simulink model "sampleModel7126_pp_1_1"  (R2018a)
settings: Solver=VariableStepAuto  StartTime=0.0  StopTime=10.0  RelTol=1e-3
undefined symbols (not defined in the file): DiscIntNeverNeededParam
libraries: simulink x367
(part 10 of 12)

== system sampleModel7126_pp_1_1/cfblk287/cfblk4 ==
  emi_718 : Inport
  Action Port : ActionPort  ActionType=then
  cfblk4 : simulink/Discrete/Transfer Fcn Lead or Lag  PoleZ=0.95  ZeroZ=0.75  ICPrevOutput=0.0  ICPrevInput=0.0  DoSatur=off
      settings: SourceProductName=Simulink  SourceProductBaseCode=SL
  emi_719 : Outport
  wires:
  emi_718/1 -> cfblk4/1
  cfblk4/1 -> emi_719/1

== system sampleModel7126_pp_1_1/cfblk287/cfblk6 ==
  emi_753 : Inport
  Action Port : ActionPort  ActionType=then
  cfblk6 : simulink/Discrete/Difference  ICPrevInput=0.0  OutMin=[]  OutMax=[]  OutDataTypeStr=double  OutputDataTypeScalingMode=double  OutDataType=fixdt(1, 16)  OutScaling=2^-10  DoSatur=off
  emi_754 : Outport
  wires:
  emi_753/1 -> cfblk6/1
  cfblk6/1 -> emi_754/1

== system sampleModel7126_pp_1_1/cfblk287/cfblk7 ==
  emi_1674 : Inport
  emi_1675 : Inport  Port=2
  Action Port : ActionPort  ActionType=then
  cfblk7 : Delay  DelayLengthSource=Input port
      settings: InputPortMap=u0,p1
  emi_1676 : Outport
  wires:
  emi_1674/1 -> cfblk7/1
  emi_1675/1 -> cfblk7/2
  cfblk7/1 -> emi_1676/1

== system sampleModel7126_pp_1_1/cfblk287/emi_1677 ==
  Action Port : ActionPort  ActionType=else
  emi_1678 : Assertion

== system sampleModel7126_pp_1_1/cfblk287/emi_720 ==
  Action Port : ActionPort  ActionType=else
  emi_721 : Assertion

== system sampleModel7126_pp_1_1/cfblk287/emi_755 ==
  Action Port : ActionPort  ActionType=else
  emi_756 : Assertion

== system sampleModel7126_pp_1_1/cfblk288/cfblk11 ==
  emi_344 : Inport
  Action Port : ActionPort  ActionType=then
  cfblk11 : simulink/Discrete/Transfer Fcn First Order  PoleZ=0.95  ICPrevOutput=0.0  DoSatur=off
      settings: SourceProductName=Simulink
  emi_345 : Outport
  wires:
  emi_344/1 -> cfblk11/1
  cfblk11/1 -> emi_345/1

== system sampleModel7126_pp_1_1/cfblk288/cfblk3 ==
  emi_1348 : Inport
  Action Port : ActionPort  ActionType=then
  cfblk3 : simulink/Continuous/PID Controller  Controller=PID  TimeDomain=Discrete-time  SampleTime=-1  IntegratorMethod=Forward Euler  FilterMethod=Forward Euler  Form=Parallel  UseFilter=on  ControllerParametersSource=internal  P=1  I=1  D=0  N=100  InitialConditionSource=internal  InitialConditionForIntegrator=0  InitialConditionForFilter=0  ExternalReset=none  LimitOutput=off  UpperSaturationLimit=inf  LowerSaturationLimit=-inf  LinearizeAsGain=off  AntiWindupMode=none  Kb=1  TrackingMode=off  Kt=1  PParamMin=[]  PParamMax=[]  IParamMin=[]  IParamMax=[]  DParamMin=[]  DParamMax=[]  NParamMin=[]  NParamMax=[]  KbParamMin=[]  KbParamMax=[]  KtParamMin=[]  KtParamMax=[]  POutMin=[]  POutMax=[]  IOutMin=[]  IOutMax=[]  DOutMin=[]  DOutMax=[]  NOutMin=[]  NOutMax=[]  KbOutMin=[]  KbOutMax=[]  KtOutMin=[]  KtOutMax=[]  IntegratorOutMin=[]  IntegratorOutMax=[]  FilterOutMin=[]  FilterOutMax=[]  SumOutMin=[]  SumOutMax=[]  SumI1OutMin=[]  SumI1OutMax=[]  SumI2OutMin=[]  SumI2OutMax=[]  SumI3OutMin=[]  SumI3OutMax=[]  SumDOutMin=[]  SumDOutMax=[]  SaturationOutMin=[]  SaturationOutMax=[]  IntegratorContinuousStateAttributes=''  IntegratorStateMustResolveToSignalObject=off  IntegratorRTWStateStorageClass=Auto  FilterContinuousStateAttributes=''  FilterStateMustResolveToSignalObject=off  FilterRTWStateStorageClass=Auto  DifferentiatorICPrevScaledInput=0  DifferentiatorOutMin=[]  DifferentiatorOutMax=[]  FilterDiffOutCoefMin=[]  FilterDiffOutCoefMax=[]  SumDenOutMin=[]  SumDenOutMax=[]  SumNumOutMin=[]  SumNumOutMax=[]  ReciprocalOutMin=[]  ReciprocalOutMax=[]  DivideOutMin=[]  DivideOutMax=[]  TunerSelectOption=Transfer Function Based (PID Tuner App)
  emi_1349 : Outport
  wires:
  emi_1348/1 -> cfblk3/1
  cfblk3/1 -> emi_1349/1

== system sampleModel7126_pp_1_1/cfblk288/emi_1350 ==
  Action Port : ActionPort  ActionType=else
  emi_1351 : Assertion

== system sampleModel7126_pp_1_1/cfblk288/emi_346 ==
  Action Port : ActionPort  ActionType=else
  emi_347 : Assertion

== system sampleModel7126_pp_1_1/cfblk289/cfblk10 ==
  cfblk1 : Inport
  cfblk12 : Inport  Port=2
  Action Port : ActionPort  ActionType=else
  cfblk10 : simulink/Discrete/Transfer Fcn Lead or Lag  PoleZ=0.95  ZeroZ=0.75  ICPrevOutput=0.0  ICPrevInput=0.0  DoSatur=off
      settings: SourceProductName=Simulink  SourceProductBaseCode=SL
  cfblk11 : Delay  DelayLengthSource=Input port
      settings: InputPortMap=u0,p1
  cfblk3 : simulink/Discrete/Transfer Fcn Lead or Lag  PoleZ=0.95  ZeroZ=0.75  ICPrevOutput=0.0  ICPrevInput=0.0  DoSatur=off
      settings: SourceProductName=Simulink  SourceProductBaseCode=SL
  cfblk4 : Subsystem  TreatAsAtomicUnit=on
  cfblk5 : Subsystem  TreatAsAtomicUnit=on
  cfblk6 : Delay  DelayLengthSource=Input port
      settings: InputPortMap=u0,p1
  cfblk7 : Subsystem  TreatAsAtomicUnit=on
  cfblk8 : simulink/Discrete/Difference  ICPrevInput=0.0  OutMin=[]  OutMax=[]  OutDataTypeStr=double  OutputDataTypeScalingMode=double  OutDataType=fixdt(1, 16)  OutScaling=2^-10  DoSatur=off
  cfblk9 : Subsystem  TreatAsAtomicUnit=on
  cyemi_{1097..1107} (11 alike) : DataTypeConversion  OutDataTypeStr=double
  emi_1407 : Subsystem  TreatAsAtomicUnit=on
  emi_{588,978,985,1409} (4 alike) : If  IfExpression=Inf <= u1  SampleTime=[1 0]
  emi_{589,979,986,1410} (4 alike) : DataTypeConversion  OutDataTypeStr=double
  emi_586 : Subsystem  TreatAsAtomicUnit=on
  emi_976 : Subsystem  TreatAsAtomicUnit=on
  emi_983 : Subsystem  TreatAsAtomicUnit=on
  cfblk2 : Outport
  wires:
  cfblk12/1 -> cyemi_1097/1, cyemi_1098/1
  cyemi_1097/1 -> cfblk10/1
  cyemi_1098/1 -> cfblk11/1
  cyemi_1099/1 -> cfblk11/2
  cfblk8/1 -> cyemi_1099/1
  cyemi_1100/1 -> cfblk3/1
  cfblk3/1 -> cyemi_1101/1
  cyemi_1103/1 -> cfblk6/1
  cfblk1/1 -> cyemi_1103/1
  cyemi_1104/1 -> cfblk6/2
  cfblk11/1 -> cyemi_1105/1, emi_979/1, emi_986/1, emi_1410/1
  cyemi_1106/1 -> cfblk8/1
  cfblk10/1 -> cyemi_1106/1
  cfblk6/1 -> cyemi_1107/1, emi_589/1
  cyemi_1107/1 -> cfblk9/1(emi_584)
  cfblk9/1(emi_585) -> cyemi_1102/1
  emi_588/1 -> cfblk9/Action
  emi_588/2 -> emi_586/Action
  emi_589/1 -> emi_588/1
  cyemi_1102/1 -> cfblk5/1(emi_974)
  cfblk5/1(emi_975) -> cyemi_1100/1
  emi_978/1 -> cfblk5/Action
  emi_978/2 -> emi_976/Action
  emi_979/1 -> emi_978/1
  cyemi_1101/1 -> cfblk4/1(emi_981)
  cfblk4/1(emi_982) -> cfblk2/1
  emi_985/1 -> cfblk4/Action
  emi_985/2 -> emi_983/Action
  emi_986/1 -> emi_985/1
  cyemi_1105/1 -> cfblk7/1(emi_1405)
  cfblk7/1(emi_1406) -> cyemi_1104/1
  emi_1409/1 -> cfblk7/Action
  emi_1409/2 -> emi_1407/Action
  emi_1410/1 -> emi_1409/1

== system sampleModel7126_pp_1_1/cfblk289/cfblk11 ==
  emi_1124 : Inport
  Action Port : ActionPort  ActionType=then
  cfblk11 : Delay
  emi_1125 : Outport
  wires:
  emi_1124/1 -> cfblk11/1
  cfblk11/1 -> emi_1125/1

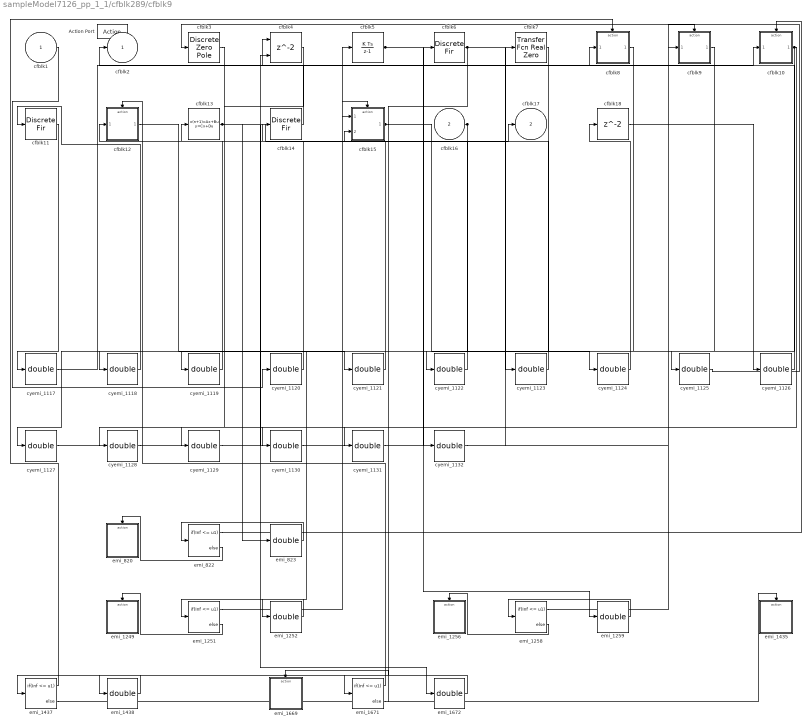
== system sampleModel7126_pp_1_1/cfblk289/cfblk9 ==
  cfblk1 : Inport
  cfblk16 : Inport  Port=2
  Action Port : ActionPort  ActionType=then
  cfblk10 : Subsystem  TreatAsAtomicUnit=on
  cfblk11 : DiscreteFir
  cfblk12 : Subsystem  TreatAsAtomicUnit=on
  cfblk13 : DiscreteStateSpace  SampleTime=-1
  cfblk14 : DiscreteFir
  cfblk15 : Subsystem  TreatAsAtomicUnit=on
  cfblk18 : Delay
  cfblk3 : DiscreteZeroPole  Poles=[0 0.5]  Gain=1  SampleTime=-1
  cfblk4 : Delay  ShowEnablePort=on
      settings: InputPortMap=u0,e6
  cfblk5 : DiscreteIntegrator  SampleTime=-1  OutDataTypeStr=double  ICPrevOutput=DiscIntNeverNeededParam  ICPrevScaledInput=DiscIntNeverNeededParam
  cfblk6 : DiscreteFir
  cfblk7 : simulink/Discrete/Transfer Fcn Real Zero  ZeroZ=0.75  ICPrevInput=0.0  DoSatur=off
      settings: SourceProductName=Simulink  SourceProductBaseCode=SL
  cfblk8 : Subsystem  TreatAsAtomicUnit=on
  cfblk9 : Subsystem  TreatAsAtomicUnit=on
  cyemi_{1117..1132} (16 alike) : DataTypeConversion  OutDataTypeStr=double
  emi_1249 : Subsystem  TreatAsAtomicUnit=on
  emi_1251 : If  IfExpression=Inf <= u1  SampleTime=[1 0]
  emi_{823,1252,1259,1438,1672} (5 alike) : DataTypeConversion  OutDataTypeStr=double
  emi_1256 : Subsystem  TreatAsAtomicUnit=on
  emi_1258 : If  IfExpression=Inf <= u1  SampleTime=[0 1]
  emi_1435 : Subsystem  TreatAsAtomicUnit=on
  emi_1437 : If  IfExpression=Inf <= u1  SampleTime=[1 0]
  emi_1669 : Subsystem  TreatAsAtomicUnit=on
  emi_1671 : If  IfExpression=Inf <= u1  SampleTime=[1 0]
  emi_820 : Subsystem  TreatAsAtomicUnit=on
  emi_822 : If  IfExpression=Inf <= u1
  cfblk2 : Outport
  cfblk17 : Outport  Port=2
  wires:
  cfblk16/1 -> cyemi_1127/1, cyemi_1130/1
  cfblk14/1 -> cfblk2/1
  cfblk13/1 -> cfblk17/1, emi_823/1, emi_1672/1
  cfblk11/1 -> cyemi_1117/1
  cyemi_1118/1 -> cfblk11/1
  cfblk7/1 -> cyemi_1118/1
  cfblk3/1 -> cyemi_1119/1
  cyemi_1120/1 -> cfblk13/1
  cfblk1/1 -> cyemi_1120/1
  cyemi_1121/1 -> cfblk14/1
  cfblk6/1 -> cyemi_1123/1, emi_1438/1
  cyemi_1124/1 -> cfblk18/1
  cyemi_1125/1 -> cfblk3/1
  cyemi_1126/1 -> cfblk4/1
  cfblk18/1 -> cyemi_1126/1
  cyemi_1127/1 -> cfblk4/2
  cyemi_1128/1 -> cfblk5/1
  cyemi_1129/1 -> cfblk6/1
  cfblk4/1 -> cyemi_1129/1
  cyemi_1130/1 -> cfblk7/1
  cfblk5/1 -> cyemi_1132/1, emi_1259/1
  cyemi_1117/1 -> cfblk10/1(emi_818)
  cfblk10/1(emi_819) -> cyemi_1131/1, emi_1252/1
  emi_822/1 -> cfblk10/Action
  emi_822/2 -> emi_820/Action
  emi_823/1 -> emi_822/1
  cyemi_1122/1 -> cfblk15/1(emi_1246)
  cyemi_1123/1 -> cfblk15/2(emi_1247)
  cfblk15/1(emi_1248) -> cyemi_1128/1, cyemi_1124/1
  emi_1251/1 -> cfblk15/Action
  emi_1251/2 -> emi_1249/Action
  emi_1252/1 -> emi_1251/1
  cyemi_1132/1 -> cfblk9/1(emi_1254)
  cfblk9/1(emi_1255) -> cyemi_1125/1
  emi_1258/1 -> cfblk9/Action
  emi_1258/2 -> emi_1256/Action
  emi_1259/1 -> emi_1258/1
  cyemi_1131/1 -> cfblk8/1(emi_1433)
  cfblk8/1(emi_1434) -> cyemi_1122/1
  emi_1437/1 -> cfblk8/Action
  emi_1437/2 -> emi_1435/Action
  emi_1438/1 -> emi_1437/1
  cyemi_1119/1 -> cfblk12/1(emi_1667)
  cfblk12/1(emi_1668) -> cyemi_1121/1
  emi_1671/1 -> cfblk12/Action
  emi_1671/2 -> emi_1669/Action
  emi_1672/1 -> emi_1671/1

== system sampleModel7126_pp_1_1/cfblk289/emi_1126 ==
  Action Port : ActionPort  ActionType=else
  emi_1127 : Assertion

== system sampleModel7126_pp_1_1/cfblk290/cfblk3 ==
  emi_1725 : Inport
  Action Port : ActionPort  ActionType=then
  cfblk3 : DiscreteTransferFcn
  emi_1726 : Outport
  wires:
  emi_1725/1 -> cfblk3/1
  cfblk3/1 -> emi_1726/1

== system sampleModel7126_pp_1_1/cfblk290/cfblk5 ==
  emi_1239 : Inport
  Action Port : ActionPort  ActionType=then
  cfblk5 : DiscreteFilter
  emi_1240 : Outport
  wires:
  emi_1239/1 -> cfblk5/1
  cfblk5/1 -> emi_1240/1

== system sampleModel7126_pp_1_1/cfblk290/cfblk6 ==
  emi_1869 : Inport
  emi_1870 : Inport  Port=2
  Action Port : ActionPort  ActionType=then
  cfblk6 : simulink/Continuous/PID Controller (2DOF)  Controller=PID  TimeDomain=Discrete-time  SampleTime=-1  IntegratorMethod=Forward Euler  FilterMethod=Forward Euler  Form=Parallel  UseFilter=on  ControllerParametersSource=internal  P=1  I=1  D=0  N=100  b=1  c=1  InitialConditionSource=internal  InitialConditionForIntegrator=0  InitialConditionForFilter=0  ExternalReset=none  LimitOutput=off  UpperSaturationLimit=inf  LowerSaturationLimit=-inf  LinearizeAsGain=off  AntiWindupMode=none  Kb=1  TrackingMode=off  Kt=1  PParamMin=[]  PParamMax=[]  IParamMin=[]  IParamMax=[]  DParamMin=[]  DParamMax=[]  NParamMin=[]  NParamMax=[]  bParamMin=[]  bParamMax=[]  cParamMin=[]  cParamMax=[]  KbParamMin=[]  KbParamMax=[]  KtParamMin=[]  KtParamMax=[]  POutMin=[]  POutMax=[]  IOutMin=[]  IOutMax=[]  DOutMin=[]  DOutMax=[]  NOutMin=[]  NOutMax=[]  bOutMin=[]  bOutMax=[]  cOutMin=[]  cOutMax=[]  KbOutMin=[]  KbOutMax=[]  KtOutMin=[]  KtOutMax=[]  IntegratorOutMin=[]  IntegratorOutMax=[]  FilterOutMin=[]  FilterOutMax=[]  SumOutMin=[]  SumOutMax=[]  Sum1OutMin=[]  Sum1OutMax=[]  Sum2OutMin=[]  Sum2OutMax=[]  Sum3OutMin=[]  Sum3OutMax=[]  SumI1OutMin=[]  SumI1OutMax=[]  SumI2OutMin=[]  SumI2OutMax=[]  SumI3OutMin=[]  SumI3OutMax=[]  SumDOutMin=[]  SumDOutMax=[]  SaturationOutMin=[]  SaturationOutMax=[]  IntegratorContinuousStateAttributes=''  IntegratorStateMustResolveToSignalObject=off  IntegratorRTWStateStorageClass=Auto  FilterContinuousStateAttributes=''  FilterStateMustResolveToSignalObject=off  FilterRTWStateStorageClass=Auto  DifferentiatorICPrevScaledInput=0  DifferentiatorOutMin=[]  DifferentiatorOutMax=[]  FilterDiffOutCoefMin=[]  FilterDiffOutCoefMax=[]  SumDenOutMin=[]  SumDenOutMax=[]  SumNumOutMin=[]  SumNumOutMax=[]  ReciprocalOutMin=[]  ReciprocalOutMax=[]  DivideOutMin=[]  DivideOutMax=[]  TunerSelectOption=Transfer Function Based (PID Tuner App)
  emi_1871 : Outport
  wires:
  emi_1869/1 -> cfblk6/1
  emi_1870/1 -> cfblk6/2
  cfblk6/1 -> emi_1871/1

== system sampleModel7126_pp_1_1/cfblk290/cfblk7 ==
  emi_1383 : Inport
  Action Port : ActionPort  ActionType=then
  cfblk7 : DiscreteFilter
  emi_1384 : Outport
  wires:
  emi_1383/1 -> cfblk7/1
  cfblk7/1 -> emi_1384/1

== system sampleModel7126_pp_1_1/cfblk290/cfblk8 ==
  emi_1152 : Inport
  Action Port : ActionPort  ActionType=then
  cfblk8 : Delay
  emi_1153 : Outport
  wires:
  emi_1152/1 -> cfblk8/1
  cfblk8/1 -> emi_1153/1

== system sampleModel7126_pp_1_1/cfblk290/emi_1154 ==
  Action Port : ActionPort  ActionType=else
  emi_1155 : Assertion

== system sampleModel7126_pp_1_1/cfblk290/emi_1241 ==
  Action Port : ActionPort  ActionType=else
  emi_1242 : Assertion

== system sampleModel7126_pp_1_1/cfblk290/emi_1385 ==
  Action Port : ActionPort  ActionType=else
  emi_1386 : Assertion

== system sampleModel7126_pp_1_1/cfblk290/emi_1727 ==
  Action Port : ActionPort  ActionType=else
  emi_1728 : Assertion

== system sampleModel7126_pp_1_1/cfblk290/emi_1872 ==
  Action Port : ActionPort  ActionType=else
  emi_1873 : Assertion

== system sampleModel7126_pp_1_1/cfblk291/cfblk6 ==
  emi_429 : Inport
  emi_430 : Inport  Port=2
  Action Port : ActionPort  ActionType=then
  cfblk6 : Delay  ShowEnablePort=on
      settings: InputPortMap=u0,e6
  emi_431 : Outport
  wires:
  emi_429/1 -> cfblk6/1
  emi_430/1 -> cfblk6/2
  cfblk6/1 -> emi_431/1

== system sampleModel7126_pp_1_1/cfblk291/emi_432 ==
  Action Port : ActionPort  ActionType=else
  emi_433 : Assertion

== system sampleModel7126_pp_1_1/cfblk292/cfblk14 ==
  cfblk1 : Inport
  Action Port : ActionPort  ActionType=then
  cfblk3 : Subsystem  TreatAsAtomicUnit=on
  cfblk4 : Subsystem  TreatAsAtomicUnit=on
  cfblk5 : simulink/Discrete/Tapped Delay  vinit=0.0  samptime=-1  NumDelays=1  DelayOrder=Oldest  includeCurrent=off
  cfblk6 : simulink/Continuous/PID Controller (2DOF)  Controller=PID  TimeDomain=Discrete-time  SampleTime=-1  IntegratorMethod=Forward Euler  FilterMethod=Forward Euler  Form=Parallel  UseFilter=on  ControllerParametersSource=internal  P=1  I=1  D=0  N=100  b=1  c=1  InitialConditionSource=internal  InitialConditionForIntegrator=0  InitialConditionForFilter=0  ExternalReset=none  LimitOutput=off  UpperSaturationLimit=inf  LowerSaturationLimit=-inf  LinearizeAsGain=off  AntiWindupMode=none  Kb=1  TrackingMode=off  Kt=1  PParamMin=[]  PParamMax=[]  IParamMin=[]  IParamMax=[]  DParamMin=[]  DParamMax=[]  NParamMin=[]  NParamMax=[]  bParamMin=[]  bParamMax=[]  cParamMin=[]  cParamMax=[]  KbParamMin=[]  KbParamMax=[]  KtParamMin=[]  KtParamMax=[]  POutMin=[]  POutMax=[]  IOutMin=[]  IOutMax=[]  DOutMin=[]  DOutMax=[]  NOutMin=[]  NOutMax=[]  bOutMin=[]  bOutMax=[]  cOutMin=[]  cOutMax=[]  KbOutMin=[]  KbOutMax=[]  KtOutMin=[]  KtOutMax=[]  IntegratorOutMin=[]  IntegratorOutMax=[]  FilterOutMin=[]  FilterOutMax=[]  SumOutMin=[]  SumOutMax=[]  Sum1OutMin=[]  Sum1OutMax=[]  Sum2OutMin=[]  Sum2OutMax=[]  Sum3OutMin=[]  Sum3OutMax=[]  SumI1OutMin=[]  SumI1OutMax=[]  SumI2OutMin=[]  SumI2OutMax=[]  SumI3OutMin=[]  SumI3OutMax=[]  SumDOutMin=[]  SumDOutMax=[]  SaturationOutMin=[]  SaturationOutMax=[]  IntegratorContinuousStateAttributes=''  IntegratorStateMustResolveToSignalObject=off  IntegratorRTWStateStorageClass=Auto  FilterContinuousStateAttributes=''  FilterStateMustResolveToSignalObject=off  FilterRTWStateStorageClass=Auto  DifferentiatorICPrevScaledInput=0  DifferentiatorOutMin=[]  DifferentiatorOutMax=[]  FilterDiffOutCoefMin=[]  FilterDiffOutCoefMax=[]  SumDenOutMin=[]  SumDenOutMax=[]  SumNumOutMin=[]  SumNumOutMax=[]  ReciprocalOutMin=[]  ReciprocalOutMax=[]  DivideOutMin=[]  DivideOutMax=[]  TunerSelectOption=Transfer Function Based (PID Tuner App)
  cfblk8 : Delay
  cfblk9 : Delay
  cyemi_{1158..1164} (7 alike) : DataTypeConversion  OutDataTypeStr=double
  emi_1428 : Subsystem  TreatAsAtomicUnit=on
  emi_1430 : If  IfExpression=Inf <= u1
  emi_1431 : DataTypeConversion  OutDataTypeStr=double
  emi_353 : Subsystem  TreatAsAtomicUnit=on
  emi_355 : If  IfExpression=Inf <= u1  SampleTime=[1 0]
  emi_356 : DataTypeConversion  OutDataTypeStr=double
  cfblk2 : Outport
  cfblk7 : Outport  Port=2
  wires:
  cfblk5/1 -> cyemi_1163/1, cyemi_1164/1
  cfblk8/1 -> cyemi_1158/1, emi_356/1, emi_1431/1
  cfblk1/1 -> cyemi_1159/1
  cyemi_1160/1 -> cfblk5/1
  cfblk6/1 -> cyemi_1160/1
  cyemi_1161/1 -> cfblk6/1
  cfblk9/1 -> cyemi_1161/1
  cyemi_1162/1 -> cfblk6/2
  cyemi_1163/1 -> cfblk8/1
  cyemi_1164/1 -> cfblk9/1
  cyemi_1159/1 -> cfblk4/1(emi_351)
  cfblk4/1(emi_352) -> cfblk7/1
  emi_355/1 -> cfblk4/Action
  emi_355/2 -> emi_353/Action
  emi_356/1 -> emi_355/1
  cyemi_1158/1 -> cfblk3/1(emi_1426)
  cfblk3/1(emi_1427) -> cyemi_1162/1, cfblk2/1
  emi_1430/1 -> cfblk3/Action
  emi_1430/2 -> emi_1428/Action
  emi_1431/1 -> emi_1430/1

== system sampleModel7126_pp_1_1/cfblk292/cfblk15 ==
  cfblk1 : Inport
  cfblk8 : Inport  Port=2
  cfblk9 : Inport  Port=3
  cfblk10 : Inport  Port=4
  Action Port : ActionPort  ActionType=else
  cfblk13 : Subsystem  TreatAsAtomicUnit=on
  cfblk3 : Subsystem  TreatAsAtomicUnit=on
  cfblk4 : UnitDelay  SampleTime=-1
  cfblk5 : Subsystem  TreatAsAtomicUnit=on
  cfblk6 : Subsystem  TreatAsAtomicUnit=on
  cfblk7 : DiscreteTransferFcn
  cyemi_{1169..1175} (7 alike) : DataTypeConversion  OutDataTypeStr=double
  emi_1414 : Subsystem  TreatAsAtomicUnit=on
  emi_1416 : If  IfExpression=0 <= u1
  emi_{458,1417,1738,1767} (4 alike) : DataTypeConversion  OutDataTypeStr=double
  emi_1735 : Subsystem  TreatAsAtomicUnit=on
  emi_1737 : If  IfExpression=0 <= u1  SampleTime=[1 0]
  emi_1764 : Subsystem  TreatAsAtomicUnit=on
  emi_1766 : If  IfExpression=0 <= u1  SampleTime=[1 0]
  emi_455 : Subsystem  TreatAsAtomicUnit=on
  emi_457 : If  IfExpression=0 <= u1
  cfblk2 : Outport
  cfblk11 : Outport  Port=2
  cfblk12 : Outport  Port=3
  wires:
  cfblk9/1 -> cfblk12/1
  cfblk8/1 -> cfblk2/1
  cfblk4/1 -> cfblk11/1
  cfblk1/1 -> cyemi_1170/1
  cyemi_1171/1 -> cfblk4/1
  cfblk7/1 -> cyemi_1171/1, emi_1738/1
  cyemi_1175/1 -> cfblk7/1
  cfblk10/1 -> cyemi_1175/1
  cyemi_1170/1 -> cfblk3/1(emi_453)
  cfblk3/1(emi_454) -> cyemi_1174/1
  emi_457/1 -> cfblk3/Action
  emi_457/2 -> emi_455/Action
  emi_458/1 -> emi_457/1
  cyemi_1169/1 -> cfblk13/1(emi_1412)
  cfblk13/1(emi_1413) -> emi_458/1, cyemi_1173/1, emi_1767/1
  emi_1416/1 -> cfblk13/Action
  emi_1416/2 -> emi_1414/Action
  emi_1417/1 -> emi_1416/1
  cyemi_1173/1 -> cfblk6/1(emi_1732)
  cyemi_1174/1 -> cfblk6/2(emi_1733)
  cfblk6/1(emi_1734) -> cyemi_1172/1
  emi_1737/1 -> cfblk6/Action
  emi_1737/2 -> emi_1735/Action
  emi_1738/1 -> emi_1737/1
  cyemi_1172/1 -> cfblk5/1(emi_1762)
  cfblk5/1(emi_1763) -> emi_1417/1, cyemi_1169/1
  emi_1766/1 -> cfblk5/Action
  emi_1766/2 -> emi_1764/Action
  emi_1767/1 -> emi_1766/1

== system sampleModel7126_pp_1_1/cfblk292/cfblk16 ==
  emi_301 : Inport
  Action Port : ActionPort  ActionType=then
  cfblk16 : Delay
  emi_302 : Outport
  wires:
  emi_301/1 -> cfblk16/1
  cfblk16/1 -> emi_302/1

== system sampleModel7126_pp_1_1/cfblk292/cfblk6 ==
  emi_1110 : Inport
  Action Port : ActionPort  ActionType=then
  cfblk6 : simulink/Discrete/Tapped Delay  vinit=0.0  samptime=-1  NumDelays=1  DelayOrder=Oldest  includeCurrent=off
  emi_1111 : Outport
  wires:
  emi_1110/1 -> cfblk6/1
  cfblk6/1 -> emi_1111/1

== system sampleModel7126_pp_1_1/cfblk292/emi_1112 ==
  Action Port : ActionPort  ActionType=else
  emi_1113 : Assertion

== system sampleModel7126_pp_1_1/cfblk292/emi_303 ==
  Action Port : ActionPort  ActionType=else
  emi_304 : Assertion

== system sampleModel7126_pp_1_1/cfblk293/cfblk10 ==
  emi_2173 : Inport
  Action Port : ActionPort  ActionType=then
  cfblk10 : Delay
  emi_2174 : Outport
  wires:
  emi_2173/1 -> cfblk10/1
  cfblk10/1 -> emi_2174/1

== system sampleModel7126_pp_1_1/cfblk293/cfblk12 ==
  emi_117 : Inport
  Action Port : ActionPort  ActionType=then
  cfblk12 : Delay
  emi_118 : Outport
  wires:
  emi_117/1 -> cfblk12/1
  cfblk12/1 -> emi_118/1

== system sampleModel7126_pp_1_1/cfblk293/cfblk4 ==
  emi_322 : Inport
  emi_323 : Inport  Port=2
  Action Port : ActionPort  ActionType=then
  cfblk4 : Delay  ShowEnablePort=on
      settings: InputPortMap=u0,e6
  emi_324 : Outport
  wires:
  emi_322/1 -> cfblk4/1
  emi_323/1 -> cfblk4/2
  cfblk4/1 -> emi_324/1

== system sampleModel7126_pp_1_1/cfblk293/cfblk8 ==
  emi_294 : Inport
  Action Port : ActionPort  ActionType=then
  cfblk8 : simulink/Discrete/Transfer Fcn First Order  PoleZ=0.95  ICPrevOutput=0.0  DoSatur=off
      settings: SourceProductName=Simulink
  emi_295 : Outport
  wires:
  emi_294/1 -> cfblk8/1
  cfblk8/1 -> emi_295/1

== system sampleModel7126_pp_1_1/cfblk293/emi_119 ==
  Action Port : ActionPort  ActionType=else
  emi_120 : Assertion

== system sampleModel7126_pp_1_1/cfblk293/emi_2175 ==
  Action Port : ActionPort  ActionType=else
  emi_2176 : Assertion

== system sampleModel7126_pp_1_1/cfblk293/emi_296 ==
  Action Port : ActionPort  ActionType=else
  emi_297 : Assertion

== system sampleModel7126_pp_1_1/cfblk293/emi_325 ==
  Action Port : ActionPort  ActionType=else
  emi_326 : Assertion

== system sampleModel7126_pp_1_1/cfblk294/cfblk3 ==
  emi_1390 : Inport
  emi_1391 : Inport  Port=2
  Action Port : ActionPort  ActionType=then
  cfblk3 : Delay  DelayLengthSource=Input port
      settings: InputPortMap=u0,p1
  emi_1392 : Outport
  wires:
  emi_1390/1 -> cfblk3/1
  emi_1391/1 -> cfblk3/2
  cfblk3/1 -> emi_1392/1

== system sampleModel7126_pp_1_1/cfblk294/cfblk7 ==
  emi_1188 : Inport
  Action Port : ActionPort  ActionType=then
  cfblk7 : Delay
  emi_1189 : Outport
  wires:
  emi_1188/1 -> cfblk7/1
  cfblk7/1 -> emi_1189/1

== system sampleModel7126_pp_1_1/cfblk294/emi_1190 ==
  Action Port : ActionPort  ActionType=else
  emi_1191 : Assertion

== system sampleModel7126_pp_1_1/cfblk294/emi_1393 ==
  Action Port : ActionPort  ActionType=else
  emi_1394 : Assertion

== system sampleModel7126_pp_1_1/cfblk295/cfblk13 ==
  cfblk1 : Inport
  cfblk15 : Inport  Port=2
  cfblk16 : Inport  Port=3
  cfblk17 : Inport  Port=4
  Action Port : ActionPort  ActionType=then
  cfblk10 : simulink/Discrete/Transfer Fcn Real Zero  ZeroZ=0.75  ICPrevInput=0.0  DoSatur=off
      settings: SourceProductName=Simulink  SourceProductBaseCode=SL
  cfblk11 : DiscreteStateSpace  SampleTime=-1
  cfblk12 : DiscreteFir
  cfblk13 : Delay  DelayLengthSource=Input port
      settings: InputPortMap=u0,p1
  cfblk14 : DiscreteFir
  cfblk3 : simulink/Continuous/PID Controller  Controller=PID  TimeDomain=Discrete-time  SampleTime=-1  IntegratorMethod=Forward Euler  FilterMethod=Forward Euler  Form=Parallel  UseFilter=on  ControllerParametersSource=internal  P=1  I=1  D=0  N=100  InitialConditionSource=internal  InitialConditionForIntegrator=0  InitialConditionForFilter=0  ExternalReset=none  LimitOutput=off  UpperSaturationLimit=inf  LowerSaturationLimit=-inf  LinearizeAsGain=off  AntiWindupMode=none  Kb=1  TrackingMode=off  Kt=1  PParamMin=[]  PParamMax=[]  IParamMin=[]  IParamMax=[]  DParamMin=[]  DParamMax=[]  NParamMin=[]  NParamMax=[]  KbParamMin=[]  KbParamMax=[]  KtParamMin=[]  KtParamMax=[]  POutMin=[]  POutMax=[]  IOutMin=[]  IOutMax=[]  DOutMin=[]  DOutMax=[]  NOutMin=[]  NOutMax=[]  KbOutMin=[]  KbOutMax=[]  KtOutMin=[]  KtOutMax=[]  IntegratorOutMin=[]  IntegratorOutMax=[]  FilterOutMin=[]  FilterOutMax=[]  SumOutMin=[]  SumOutMax=[]  SumI1OutMin=[]  SumI1OutMax=[]  SumI2OutMin=[]  SumI2OutMax=[]  SumI3OutMin=[]  SumI3OutMax=[]  SumDOutMin=[]  SumDOutMax=[]  SaturationOutMin=[]  SaturationOutMax=[]  IntegratorContinuousStateAttributes=''  IntegratorStateMustResolveToSignalObject=off  IntegratorRTWStateStorageClass=Auto  FilterContinuousStateAttributes=''  FilterStateMustResolveToSignalObject=off  FilterRTWStateStorageClass=Auto  DifferentiatorICPrevScaledInput=0  DifferentiatorOutMin=[]  DifferentiatorOutMax=[]  FilterDiffOutCoefMin=[]  FilterDiffOutCoefMax=[]  SumDenOutMin=[]  SumDenOutMax=[]  SumNumOutMin=[]  SumNumOutMax=[]  ReciprocalOutMin=[]  ReciprocalOutMax=[]  DivideOutMin=[]  DivideOutMax=[]  TunerSelectOption=Transfer Function Based (PID Tuner App)
  cfblk4 : simulink/Discrete/Tapped Delay  vinit=0.0  samptime=-1  NumDelays=1  DelayOrder=Oldest  includeCurrent=off
  cfblk5 : Subsystem  TreatAsAtomicUnit=on
  cfblk6 : simulink/Discrete/Difference  ICPrevInput=0.0  OutMin=[]  OutMax=[]  OutDataTypeStr=double  OutputDataTypeScalingMode=double  OutDataType=fixdt(1, 16)  OutScaling=2^-10  DoSatur=off
  cfblk7 : simulink/Continuous/PID Controller (2DOF)  Controller=PID  TimeDomain=Discrete-time  SampleTime=-1  IntegratorMethod=Forward Euler  FilterMethod=Forward Euler  Form=Parallel  UseFilter=on  ControllerParametersSource=internal  P=1  I=1  D=0  N=100  b=1  c=1  InitialConditionSource=internal  InitialConditionForIntegrator=0  InitialConditionForFilter=0  ExternalReset=none  LimitOutput=off  UpperSaturationLimit=inf  LowerSaturationLimit=-inf  LinearizeAsGain=off  AntiWindupMode=none  Kb=1  TrackingMode=off  Kt=1  PParamMin=[]  PParamMax=[]  IParamMin=[]  IParamMax=[]  DParamMin=[]  DParamMax=[]  NParamMin=[]  NParamMax=[]  bParamMin=[]  bParamMax=[]  cParamMin=[]  cParamMax=[]  KbParamMin=[]  KbParamMax=[]  KtParamMin=[]  KtParamMax=[]  POutMin=[]  POutMax=[]  IOutMin=[]  IOutMax=[]  DOutMin=[]  DOutMax=[]  NOutMin=[]  NOutMax=[]  bOutMin=[]  bOutMax=[]  cOutMin=[]  cOutMax=[]  KbOutMin=[]  KbOutMax=[]  KtOutMin=[]  KtOutMax=[]  IntegratorOutMin=[]  IntegratorOutMax=[]  FilterOutMin=[]  FilterOutMax=[]  SumOutMin=[]  SumOutMax=[]  Sum1OutMin=[]  Sum1OutMax=[]  Sum2OutMin=[]  Sum2OutMax=[]  Sum3OutMin=[]  Sum3OutMax=[]  SumI1OutMin=[]  SumI1OutMax=[]  SumI2OutMin=[]  SumI2OutMax=[]  SumI3OutMin=[]  SumI3OutMax=[]  SumDOutMin=[]  SumDOutMax=[]  SaturationOutMin=[]  SaturationOutMax=[]  IntegratorContinuousStateAttributes=''  IntegratorStateMustResolveToSignalObject=off  IntegratorRTWStateStorageClass=Auto  FilterContinuousStateAttributes=''  FilterStateMustResolveToSignalObject=off  FilterRTWStateStorageClass=Auto  DifferentiatorICPrevScaledInput=0  DifferentiatorOutMin=[]  DifferentiatorOutMax=[]  FilterDiffOutCoefMin=[]  FilterDiffOutCoefMax=[]  SumDenOutMin=[]  SumDenOutMax=[]  SumNumOutMin=[]  SumNumOutMax=[]  ReciprocalOutMin=[]  ReciprocalOutMax=[]  DivideOutMin=[]  DivideOutMax=[]  TunerSelectOption=Transfer Function Based (PID Tuner App)
  cfblk8 : simulink/Discrete/Transfer Fcn Real Zero  ZeroZ=0.75  ICPrevInput=0.0  DoSatur=off
      settings: SourceProductName=Simulink  SourceProductBaseCode=SL
  cfblk9 : simulink/Discrete/Tapped Delay  vinit=0.0  samptime=-1  NumDelays=1  DelayOrder=Oldest  includeCurrent=off
  cyemi_{1224..1237} (14 alike) : DataTypeConversion  OutDataTypeStr=double
  emi_990 : Subsystem  TreatAsAtomicUnit=on
  emi_992 : If  IfExpression=Inf <= u1  SampleTime=[1 0]
  emi_993 : DataTypeConversion  OutDataTypeStr=double
  cfblk2 : Outport
  wires:
  cfblk4/1 -> cfblk2/1
  cyemi_1224/1 -> cfblk10/1
  cfblk1/1 -> cyemi_1224/1
  cyemi_1225/1 -> cfblk11/1
  cfblk14/1 -> cyemi_1225/1
  cyemi_1226/1 -> cfblk12/1
  cfblk11/1 -> cyemi_1226/1
  cyemi_1227/1 -> cfblk13/1
  cfblk17/1 -> cyemi_1227/1
  cyemi_1228/1 -> cfblk13/2
  cyemi_1229/1 -> cfblk14/1
  cfblk16/1 -> cyemi_1229/1
  cyemi_1230/1 -> cfblk3/1
  cfblk10/1 -> cyemi_1230/1
  cyemi_1231/1 -> cfblk4/1
  cfblk8/1 -> cyemi_1231/1
  cfblk15/1 -> cyemi_1232/1
  cyemi_1233/1 -> cfblk6/1
  cfblk9/1 -> cyemi_1233/1
  cyemi_1234/1 -> cfblk7/1
  cfblk6/1 -> cyemi_1234/1
  cyemi_1235/1 -> cfblk7/2
  cfblk13/1 -> cyemi_1235/1, emi_993/1
  cyemi_1236/1 -> cfblk8/1
  cfblk7/1 -> cyemi_1236/1
  cyemi_1237/1 -> cfblk9/1
  cfblk12/1 -> cyemi_1237/1
  cyemi_1232/1 -> cfblk5/1(emi_988)
  cfblk5/1(emi_989) -> cyemi_1228/1
  emi_992/1 -> cfblk5/Action
  emi_992/2 -> emi_990/Action
  emi_993/1 -> emi_992/1

== system sampleModel7126_pp_1_1/cfblk295/cfblk14 ==
  cfblk1 : Inport
  cfblk14 : Inport  Port=2
  cfblk15 : Inport  Port=3
  Action Port : ActionPort  ActionType=else
  cfblk10 : UnitDelay  SampleTime=-1
  cfblk11 : Subsystem  TreatAsAtomicUnit=on
  cfblk12 : Subsystem  TreatAsAtomicUnit=on
  cfblk13 : DiscreteZeroPole  Poles=[0 0.5]  Gain=1  SampleTime=-1
  cfblk16 : Delay
  cfblk3 : DiscreteStateSpace  SampleTime=-1
  cfblk4 : simulink/Discrete/Difference  ICPrevInput=0.0  OutMin=[]  OutMax=[]  OutDataTypeStr=double  OutputDataTypeScalingMode=double  OutDataType=fixdt(1, 16)  OutScaling=2^-10  DoSatur=off
  cfblk5 : simulink/Continuous/PID Controller (2DOF)  Controller=PID  TimeDomain=Discrete-time  SampleTime=-1  IntegratorMethod=Forward Euler  FilterMethod=Forward Euler  Form=Parallel  UseFilter=on  ControllerParametersSource=internal  P=1  I=1  D=0  N=100  b=1  c=1  InitialConditionSource=internal  InitialConditionForIntegrator=0  InitialConditionForFilter=0  ExternalReset=none  LimitOutput=off  UpperSaturationLimit=inf  LowerSaturationLimit=-inf  LinearizeAsGain=off  AntiWindupMode=none  Kb=1  TrackingMode=off  Kt=1  PParamMin=[]  PParamMax=[]  IParamMin=[]  IParamMax=[]  DParamMin=[]  DParamMax=[]  NParamMin=[]  NParamMax=[]  bParamMin=[]  bParamMax=[]  cParamMin=[]  cParamMax=[]  KbParamMin=[]  KbParamMax=[]  KtParamMin=[]  KtParamMax=[]  POutMin=[]  POutMax=[]  IOutMin=[]  IOutMax=[]  DOutMin=[]  DOutMax=[]  NOutMin=[]  NOutMax=[]  bOutMin=[]  bOutMax=[]  cOutMin=[]  cOutMax=[]  KbOutMin=[]  KbOutMax=[]  KtOutMin=[]  KtOutMax=[]  IntegratorOutMin=[]  IntegratorOutMax=[]  FilterOutMin=[]  FilterOutMax=[]  SumOutMin=[]  SumOutMax=[]  Sum1OutMin=[]  Sum1OutMax=[]  Sum2OutMin=[]  Sum2OutMax=[]  Sum3OutMin=[]  Sum3OutMax=[]  SumI1OutMin=[]  SumI1OutMax=[]  SumI2OutMin=[]  SumI2OutMax=[]  SumI3OutMin=[]  SumI3OutMax=[]  SumDOutMin=[]  SumDOutMax=[]  SaturationOutMin=[]  SaturationOutMax=[]  IntegratorContinuousStateAttributes=''  IntegratorStateMustResolveToSignalObject=off  IntegratorRTWStateStorageClass=Auto  FilterContinuousStateAttributes=''  FilterStateMustResolveToSignalObject=off  FilterRTWStateStorageClass=Auto  DifferentiatorICPrevScaledInput=0  DifferentiatorOutMin=[]  DifferentiatorOutMax=[]  FilterDiffOutCoefMin=[]  FilterDiffOutCoefMax=[]  SumDenOutMin=[]  SumDenOutMax=[]  SumNumOutMin=[]  SumNumOutMax=[]  ReciprocalOutMin=[]  ReciprocalOutMax=[]  DivideOutMin=[]  DivideOutMax=[]  TunerSelectOption=Transfer Function Based (PID Tuner App)
  cfblk6 : Subsystem  TreatAsAtomicUnit=on
  cfblk7 : Subsystem  TreatAsAtomicUnit=on
  cfblk8 : simulink/Discrete/Transfer Fcn Real Zero  ZeroZ=0.75  ICPrevInput=0.0  DoSatur=off
      settings: SourceProductName=Simulink  SourceProductBaseCode=SL
  cfblk9 : simulink/Continuous/PID Controller (2DOF)  Controller=PID  TimeDomain=Discrete-time  SampleTime=-1  IntegratorMethod=Forward Euler  FilterMethod=Forward Euler  Form=Parallel  UseFilter=on  ControllerParametersSource=internal  P=1  I=1  D=0  N=100  b=1  c=1  InitialConditionSource=internal  InitialConditionForIntegrator=0  InitialConditionForFilter=0  ExternalReset=none  LimitOutput=off  UpperSaturationLimit=inf  LowerSaturationLimit=-inf  LinearizeAsGain=off  AntiWindupMode=none  Kb=1  TrackingMode=off  Kt=1  PParamMin=[]  PParamMax=[]  IParamMin=[]  IParamMax=[]  DParamMin=[]  DParamMax=[]  NParamMin=[]  NParamMax=[]  bParamMin=[]  bParamMax=[]  cParamMin=[]  cParamMax=[]  KbParamMin=[]  KbParamMax=[]  KtParamMin=[]  KtParamMax=[]  POutMin=[]  POutMax=[]  IOutMin=[]  IOutMax=[]  DOutMin=[]  DOutMax=[]  NOutMin=[]  NOutMax=[]  bOutMin=[]  bOutMax=[]  cOutMin=[]  cOutMax=[]  KbOutMin=[]  KbOutMax=[]  KtOutMin=[]  KtOutMax=[]  IntegratorOutMin=[]  IntegratorOutMax=[]  FilterOutMin=[]  FilterOutMax=[]  SumOutMin=[]  SumOutMax=[]  Sum1OutMin=[]  Sum1OutMax=[]  Sum2OutMin=[]  Sum2OutMax=[]  Sum3OutMin=[]  Sum3OutMax=[]  SumI1OutMin=[]  SumI1OutMax=[]  SumI2OutMin=[]  SumI2OutMax=[]  SumI3OutMin=[]  SumI3OutMax=[]  SumDOutMin=[]  SumDOutMax=[]  SaturationOutMin=[]  SaturationOutMax=[]  IntegratorContinuousStateAttributes=''  IntegratorStateMustResolveToSignalObject=off  IntegratorRTWStateStorageClass=Auto  FilterContinuousStateAttributes=''  FilterStateMustResolveToSignalObject=off  FilterRTWStateStorageClass=Auto  DifferentiatorICPrevScaledInput=0  DifferentiatorOutMin=[]  DifferentiatorOutMax=[]  FilterDiffOutCoefMin=[]  FilterDiffOutCoefMax=[]  SumDenOutMin=[]  SumDenOutMax=[]  SumNumOutMin=[]  SumNumOutMax=[]  ReciprocalOutMin=[]  ReciprocalOutMax=[]  DivideOutMin=[]  DivideOutMax=[]  TunerSelectOption=Transfer Function Based (PID Tuner App)
  cyemi_{1241..1254} (14 alike) : DataTypeConversion  OutDataTypeStr=double
  emi_1212 : Subsystem  TreatAsAtomicUnit=on
  emi_{426,1214,1366,1803} (4 alike) : If  IfExpression=Inf <= u1  SampleTime=[1 0]
  emi_{427,1215,1367,1804} (4 alike) : DataTypeConversion  OutDataTypeStr=double
  emi_1364 : Subsystem  TreatAsAtomicUnit=on
  emi_1801 : Subsystem  TreatAsAtomicUnit=on
  emi_424 : Subsystem  TreatAsAtomicUnit=on
  cfblk2 : Outport
  wires:
  cyemi_1241/1 -> cfblk10/1
  cfblk8/1 -> cyemi_1241/1
  cfblk13/1 -> cyemi_1242/1, emi_427/1, emi_1804/1
  cyemi_1244/1 -> cfblk13/1
  cfblk4/1 -> cyemi_1244/1
  cyemi_1245/1 -> cfblk16/1
  cfblk10/1 -> cyemi_1245/1, emi_1215/1
  cyemi_1246/1 -> cfblk3/1
  cfblk16/1 -> cyemi_1246/1
  cyemi_1247/1 -> cfblk4/1
  cfblk5/1 -> cyemi_1247/1
  cyemi_1248/1 -> cfblk5/1
  cyemi_1249/1 -> cfblk5/2
  cfblk15/1 -> cyemi_1250/1
  cfblk1/1 -> cyemi_1251/1
  cyemi_1252/1 -> cfblk8/1
  cfblk9/1 -> cyemi_1252/1
  cyemi_1253/1 -> cfblk9/1
  cfblk3/1 -> cyemi_1253/1, emi_1367/1
  cyemi_1254/1 -> cfblk9/2
  cfblk14/1 -> cyemi_1254/1
  cyemi_1242/1 -> cfblk11/1(emi_422)
  cfblk11/1(emi_423) -> cfblk2/1
  emi_426/1 -> cfblk11/Action
  emi_426/2 -> emi_424/Action
  emi_427/1 -> emi_426/1
  cyemi_1243/1 -> cfblk12/1(emi_1210)
  cfblk12/1(emi_1211) -> cyemi_1249/1
  emi_1214/1 -> cfblk12/Action
  emi_1214/2 -> emi_1212/Action
  emi_1215/1 -> emi_1214/1
  cyemi_1250/1 -> cfblk6/1(emi_1362)
  cfblk6/1(emi_1363) -> cyemi_1243/1
  emi_1366/1 -> cfblk6/Action
  emi_1366/2 -> emi_1364/Action
  emi_1367/1 -> emi_1366/1
  cyemi_1251/1 -> cfblk7/1(emi_1799)
  cfblk7/1(emi_1800) -> cyemi_1248/1
  emi_1803/1 -> cfblk7/Action
  emi_1803/2 -> emi_1801/Action
  emi_1804/1 -> emi_1803/1

== system sampleModel7126_pp_1_1/cfblk295/cfblk15 ==
  emi_704 : Inport
  Action Port : ActionPort  ActionType=then
  cfblk15 : Delay
  emi_705 : Outport
  wires:
  emi_704/1 -> cfblk15/1
  cfblk15/1 -> emi_705/1

== system sampleModel7126_pp_1_1/cfblk295/cfblk16 ==
  emi_36 : Inport
  Action Port : ActionPort  ActionType=then
  cfblk16 : Delay
  emi_37 : Outport
  wires:
  emi_36/1 -> cfblk16/1
  cfblk16/1 -> emi_37/1

== system sampleModel7126_pp_1_1/cfblk295/emi_38 ==
  Action Port : ActionPort  ActionType=else
  emi_39 : Assertion

== system sampleModel7126_pp_1_1/cfblk295/emi_706 ==
  Action Port : ActionPort  ActionType=else
  emi_707 : Assertion

== system sampleModel7126_pp_1_1/cfblk296/cfblk10 ==
  emi_29 : Inport
  Action Port : ActionPort  ActionType=then
  cfblk10 : simulink/Discrete/Transfer Fcn First Order  PoleZ=0.95  ICPrevOutput=0.0  DoSatur=off
      settings: SourceProductName=Simulink
  emi_30 : Outport
  wires:
  emi_29/1 -> cfblk10/1
  cfblk10/1 -> emi_30/1

== system sampleModel7126_pp_1_1/cfblk296/cfblk11 ==
  emi_223 : Inport
  Action Port : ActionPort  ActionType=then
  cfblk11 : simulink/Continuous/PID Controller  Controller=PID  TimeDomain=Discrete-time  SampleTime=-1  IntegratorMethod=Forward Euler  FilterMethod=Forward Euler  Form=Parallel  UseFilter=on  ControllerParametersSource=internal  P=1  I=1  D=0  N=100  InitialConditionSource=internal  InitialConditionForIntegrator=0  InitialConditionForFilter=0  ExternalReset=none  LimitOutput=off  UpperSaturationLimit=inf  LowerSaturationLimit=-inf  LinearizeAsGain=off  AntiWindupMode=none  Kb=1  TrackingMode=off  Kt=1  PParamMin=[]  PParamMax=[]  IParamMin=[]  IParamMax=[]  DParamMin=[]  DParamMax=[]  NParamMin=[]  NParamMax=[]  KbParamMin=[]  KbParamMax=[]  KtParamMin=[]  KtParamMax=[]  POutMin=[]  POutMax=[]  IOutMin=[]  IOutMax=[]  DOutMin=[]  DOutMax=[]  NOutMin=[]  NOutMax=[]  KbOutMin=[]  KbOutMax=[]  KtOutMin=[]  KtOutMax=[]  IntegratorOutMin=[]  IntegratorOutMax=[]  FilterOutMin=[]  FilterOutMax=[]  SumOutMin=[]  SumOutMax=[]  SumI1OutMin=[]  SumI1OutMax=[]  SumI2OutMin=[]  SumI2OutMax=[]  SumI3OutMin=[]  SumI3OutMax=[]  SumDOutMin=[]  SumDOutMax=[]  SaturationOutMin=[]  SaturationOutMax=[]  IntegratorContinuousStateAttributes=''  IntegratorStateMustResolveToSignalObject=off  IntegratorRTWStateStorageClass=Auto  FilterContinuousStateAttributes=''  FilterStateMustResolveToSignalObject=off  FilterRTWStateStorageClass=Auto  DifferentiatorICPrevScaledInput=0  DifferentiatorOutMin=[]  DifferentiatorOutMax=[]  FilterDiffOutCoefMin=[]  FilterDiffOutCoefMax=[]  SumDenOutMin=[]  SumDenOutMax=[]  SumNumOutMin=[]  SumNumOutMax=[]  ReciprocalOutMin=[]  ReciprocalOutMax=[]  DivideOutMin=[]  DivideOutMax=[]  TunerSelectOption=Transfer Function Based (PID Tuner App)
  emi_224 : Outport
  wires:
  emi_223/1 -> cfblk11/1
  cfblk11/1 -> emi_224/1

== system sampleModel7126_pp_1_1/cfblk296/cfblk19 ==
  emi_22 : Inport
  Action Port : ActionPort  ActionType=then
  cfblk19 : Delay
  emi_23 : Outport
  wires:
  emi_22/1 -> cfblk19/1
  cfblk19/1 -> emi_23/1

== system sampleModel7126_pp_1_1/cfblk296/cfblk3 ==
  emi_1754 : Inport
  emi_1755 : Inport  Port=2
  Action Port : ActionPort  ActionType=then
  cfblk3 : Delay  ShowEnablePort=on
      settings: InputPortMap=u0,e6
  emi_1756 : Outport
  wires:
  emi_1754/1 -> cfblk3/1
  emi_1755/1 -> cfblk3/2
  cfblk3/1 -> emi_1756/1

== system sampleModel7126_pp_1_1/cfblk296/cfblk6 ==
  emi_445 : Inport
  emi_446 : Inport  Port=2
  Action Port : ActionPort  ActionType=then
  cfblk6 : Delay  ShowEnablePort=on
      settings: InputPortMap=u0,e6
  emi_447 : Outport
  wires:
  emi_445/1 -> cfblk6/1
  emi_446/1 -> cfblk6/2
  cfblk6/1 -> emi_447/1

== system sampleModel7126_pp_1_1/cfblk296/cfblk7 ==
  emi_159 : Inport
  Action Port : ActionPort  ActionType=then
  cfblk7 : simulink/Discrete/Tapped Delay  vinit=0.0  samptime=-1  NumDelays=1  DelayOrder=Oldest  includeCurrent=off
  emi_160 : Outport
  wires:
  emi_159/1 -> cfblk7/1
  cfblk7/1 -> emi_160/1

== system sampleModel7126_pp_1_1/cfblk296/cfblk8 ==
  emi_1511 : Inport
  Action Port : ActionPort  ActionType=then
  cfblk8 : simulink/Discrete/Tapped Delay  vinit=0.0  samptime=-1  NumDelays=1  DelayOrder=Oldest  includeCurrent=off
  emi_1512 : Outport
  wires:
  emi_1511/1 -> cfblk8/1
  cfblk8/1 -> emi_1512/1

== system sampleModel7126_pp_1_1/cfblk296/cfblk9 ==
  emi_1625 : Inport
  Action Port : ActionPort  ActionType=then
  cfblk9 : DiscreteFilter
  emi_1626 : Outport
  wires:
  emi_1625/1 -> cfblk9/1
  cfblk9/1 -> emi_1626/1

== system sampleModel7126_pp_1_1/cfblk296/emi_1513 ==
  Action Port : ActionPort  ActionType=else
  emi_1514 : Assertion

== system sampleModel7126_pp_1_1/cfblk296/emi_161 ==
  Action Port : ActionPort  ActionType=else
  emi_162 : Assertion

== system sampleModel7126_pp_1_1/cfblk296/emi_1627 ==
  Action Port : ActionPort  ActionType=else
  emi_1628 : Assertion

== system sampleModel7126_pp_1_1/cfblk296/emi_1757 ==
  Action Port : ActionPort  ActionType=else
  emi_1758 : Assertion

== system sampleModel7126_pp_1_1/cfblk296/emi_225 ==
  Action Port : ActionPort  ActionType=else
  emi_226 : Assertion

== system sampleModel7126_pp_1_1/cfblk296/emi_24 ==
  Action Port : ActionPort  ActionType=else
  emi_25 : Assertion

== system sampleModel7126_pp_1_1/cfblk296/emi_31 ==
  Action Port : ActionPort  ActionType=else
  emi_32 : Assertion

== system sampleModel7126_pp_1_1/cfblk296/emi_448 ==
  Action Port : ActionPort  ActionType=else
  emi_449 : Assertion

== system sampleModel7126_pp_1_1/cfblk297/cfblk7 ==
  emi_2029 : Inport
  emi_2030 : Inport  Port=2
  Action Port : ActionPort  ActionType=then
  cfblk7 : simulink/Continuous/PID Controller (2DOF)  Controller=PID  TimeDomain=Discrete-time  SampleTime=-1  IntegratorMethod=Forward Euler  FilterMethod=Forward Euler  Form=Parallel  UseFilter=on  ControllerParametersSource=internal  P=1  I=1  D=0  N=100  b=1  c=1  InitialConditionSource=internal  InitialConditionForIntegrator=0  InitialConditionForFilter=0  ExternalReset=none  LimitOutput=off  UpperSaturationLimit=inf  LowerSaturationLimit=-inf  LinearizeAsGain=off  AntiWindupMode=none  Kb=1  TrackingMode=off  Kt=1  PParamMin=[]  PParamMax=[]  IParamMin=[]  IParamMax=[]  DParamMin=[]  DParamMax=[]  NParamMin=[]  NParamMax=[]  bParamMin=[]  bParamMax=[]  cParamMin=[]  cParamMax=[]  KbParamMin=[]  KbParamMax=[]  KtParamMin=[]  KtParamMax=[]  POutMin=[]  POutMax=[]  IOutMin=[]  IOutMax=[]  DOutMin=[]  DOutMax=[]  NOutMin=[]  NOutMax=[]  bOutMin=[]  bOutMax=[]  cOutMin=[]  cOutMax=[]  KbOutMin=[]  KbOutMax=[]  KtOutMin=[]  KtOutMax=[]  IntegratorOutMin=[]  IntegratorOutMax=[]  FilterOutMin=[]  FilterOutMax=[]  SumOutMin=[]  SumOutMax=[]  Sum1OutMin=[]  Sum1OutMax=[]  Sum2OutMin=[]  Sum2OutMax=[]  Sum3OutMin=[]  Sum3OutMax=[]  SumI1OutMin=[]  SumI1OutMax=[]  SumI2OutMin=[]  SumI2OutMax=[]  SumI3OutMin=[]  SumI3OutMax=[]  SumDOutMin=[]  SumDOutMax=[]  SaturationOutMin=[]  SaturationOutMax=[]  IntegratorContinuousStateAttributes=''  IntegratorStateMustResolveToSignalObject=off  IntegratorRTWStateStorageClass=Auto  FilterContinuousStateAttributes=''  FilterStateMustResolveToSignalObject=off  FilterRTWStateStorageClass=Auto  DifferentiatorICPrevScaledInput=0  DifferentiatorOutMin=[]  DifferentiatorOutMax=[]  FilterDiffOutCoefMin=[]  FilterDiffOutCoefMax=[]  SumDenOutMin=[]  SumDenOutMax=[]  SumNumOutMin=[]  SumNumOutMax=[]  ReciprocalOutMin=[]  ReciprocalOutMax=[]  DivideOutMin=[]  DivideOutMax=[]  TunerSelectOption=Transfer Function Based (PID Tuner App)
  emi_2031 : Outport
  wires:
  emi_2029/1 -> cfblk7/1
  emi_2030/1 -> cfblk7/2
  cfblk7/1 -> emi_2031/1

== system sampleModel7126_pp_1_1/cfblk297/emi_2032 ==
  Action Port : ActionPort  ActionType=else
  emi_2033 : Assertion

== system sampleModel7126_pp_1_1/cfblk298/cfblk15 ==
  cfblk1 : Inport
  cfblk14 : Inport  Port=2
  Action Port : ActionPort  ActionType=then
  cfblk10 : DiscreteIntegrator  SampleTime=-1  OutDataTypeStr=double  ICPrevOutput=DiscIntNeverNeededParam  ICPrevScaledInput=DiscIntNeverNeededParam
  cfblk11 : DiscreteZeroPole  Poles=[0 0.5]  Gain=1  SampleTime=-1
  cfblk12 : Delay  ShowEnablePort=on
      settings: InputPortMap=u0,e6
  cfblk13 : DiscreteIntegrator  SampleTime=-1  OutDataTypeStr=double  ICPrevOutput=DiscIntNeverNeededParam  ICPrevScaledInput=DiscIntNeverNeededParam
  cfblk16 : Delay
  cfblk3 : DiscreteZeroPole  Poles=[0 0.5]  Gain=1  SampleTime=-1
  cfblk4 : Subsystem  TreatAsAtomicUnit=on
  cfblk5 : Subsystem  TreatAsAtomicUnit=on
  cfblk6 : simulink/Continuous/PID Controller  Controller=PID  TimeDomain=Discrete-time  SampleTime=-1  IntegratorMethod=Forward Euler  FilterMethod=Forward Euler  Form=Parallel  UseFilter=on  ControllerParametersSource=internal  P=1  I=1  D=0  N=100  InitialConditionSource=internal  InitialConditionForIntegrator=0  InitialConditionForFilter=0  ExternalReset=none  LimitOutput=off  UpperSaturationLimit=inf  LowerSaturationLimit=-inf  LinearizeAsGain=off  AntiWindupMode=none  Kb=1  TrackingMode=off  Kt=1  PParamMin=[]  PParamMax=[]  IParamMin=[]  IParamMax=[]  DParamMin=[]  DParamMax=[]  NParamMin=[]  NParamMax=[]  KbParamMin=[]  KbParamMax=[]  KtParamMin=[]  KtParamMax=[]  POutMin=[]  POutMax=[]  IOutMin=[]  IOutMax=[]  DOutMin=[]  DOutMax=[]  NOutMin=[]  NOutMax=[]  KbOutMin=[]  KbOutMax=[]  KtOutMin=[]  KtOutMax=[]  IntegratorOutMin=[]  IntegratorOutMax=[]  FilterOutMin=[]  FilterOutMax=[]  SumOutMin=[]  SumOutMax=[]  SumI1OutMin=[]  SumI1OutMax=[]  SumI2OutMin=[]  SumI2OutMax=[]  SumI3OutMin=[]  SumI3OutMax=[]  SumDOutMin=[]  SumDOutMax=[]  SaturationOutMin=[]  SaturationOutMax=[]  IntegratorContinuousStateAttributes=''  IntegratorStateMustResolveToSignalObject=off  IntegratorRTWStateStorageClass=Auto  FilterContinuousStateAttributes=''  FilterStateMustResolveToSignalObject=off  FilterRTWStateStorageClass=Auto  DifferentiatorICPrevScaledInput=0  DifferentiatorOutMin=[]  DifferentiatorOutMax=[]  FilterDiffOutCoefMin=[]  FilterDiffOutCoefMax=[]  SumDenOutMin=[]  SumDenOutMax=[]  SumNumOutMin=[]  SumNumOutMax=[]  ReciprocalOutMin=[]  ReciprocalOutMax=[]  DivideOutMin=[]  DivideOutMax=[]  TunerSelectOption=Transfer Function Based (PID Tuner App)
  cfblk7 : Subsystem  TreatAsAtomicUnit=on
  cfblk8 : UnitDelay  SampleTime=-1
  cfblk9 : Subsystem  TreatAsAtomicUnit=on
  cyemi_{1301..1313} (13 alike) : DataTypeConversion  OutDataTypeStr=double
  emi_1684 : Subsystem  TreatAsAtomicUnit=on
  emi_1686 : If  IfExpression=Inf <= u1  SampleTime=[1 0]
  emi_{638,1687,2027,2071} (4 alike) : DataTypeConversion  OutDataTypeStr=double
  emi_2024 : Subsystem  TreatAsAtomicUnit=on
  emi_2026 : If  IfExpression=Inf <= u1  SampleTime=[0.1 0]
  emi_2068 : Subsystem  TreatAsAtomicUnit=on
  emi_2070 : If  IfExpression=Inf <= u1  SampleTime=[1 0]
  emi_635 : Subsystem  TreatAsAtomicUnit=on
  emi_637 : If  IfExpression=Inf <= u1  SampleTime=[1 0]
  cfblk2 : Outport
  cfblk15 : Outport  Port=2
  wires:
  cfblk8/1 -> cyemi_1304/1, cyemi_1306/1
  cfblk13/1 -> cfblk15/1, emi_1687/1
  cyemi_1301/1 -> cfblk10/1
  cfblk14/1 -> cyemi_1301/1
  cyemi_1302/1 -> cfblk11/1
  cfblk10/1 -> cyemi_1302/1
  cyemi_1303/1 -> cfblk12/1
  cfblk3/1 -> cyemi_1303/1
  cyemi_1304/1 -> cfblk12/2
  cyemi_1305/1 -> cfblk13/1
  cyemi_1306/1 -> cfblk16/1
  cyemi_1307/1 -> cfblk3/1
  cfblk11/1 -> cyemi_1307/1, emi_638/1, emi_2027/1
  cfblk6/1 -> cyemi_1308/1
  cfblk16/1 -> cyemi_1309/1
  cyemi_1310/1 -> cfblk6/1
  cfblk1/1 -> cyemi_1310/1
  cyemi_1312/1 -> cfblk8/1
  cfblk12/1 -> cyemi_1313/1
  cyemi_1309/1 -> cfblk5/1(emi_633)
  cfblk5/1(emi_634) -> cyemi_1312/1
  emi_637/1 -> cfblk5/Action
  emi_637/2 -> emi_635/Action
  emi_638/1 -> emi_637/1
  cyemi_1308/1 -> cfblk4/1(emi_1682)
  cfblk4/1(emi_1683) -> cyemi_1305/1, emi_2071/1
  emi_1686/1 -> cfblk4/Action
  emi_1686/2 -> emi_1684/Action
  emi_1687/1 -> emi_1686/1
  cyemi_1313/1 -> cfblk9/1(emi_2022)
  cfblk9/1(emi_2023) -> cyemi_1311/1
  emi_2026/1 -> cfblk9/Action
  emi_2026/2 -> emi_2024/Action
  emi_2027/1 -> emi_2026/1
  cyemi_1311/1 -> cfblk7/1(emi_2066)
  cfblk7/1(emi_2067) -> cfblk2/1
  emi_2070/1 -> cfblk7/Action
  emi_2070/2 -> emi_2068/Action
  emi_2071/1 -> emi_2070/1
